simulink model "f1simlu"  (R2026a)
settings: Solver=VariableStepAuto  StopTime=30
values from neighbouring files (symbols this model uses):
  A = 2.2    [vehicleparameter.m]
  Cd = 0.32    [vehicleparameter.m]
  F_drive = 4000    [vehicleparameter.m]
  m = masses(k)    [laptimestudy.m]    (also in runsensitivitystudy 2.m; vehicleparameter.m = 800)
  rho = 1.225    [vehicleparameter.m]
  theta = deg2rad(theta_deg(k))    [roadgradientstudy.m]    (also in vehicleparameter.m = 0)
settings Model: Creator=manoj  LastModifiedBy=manoj

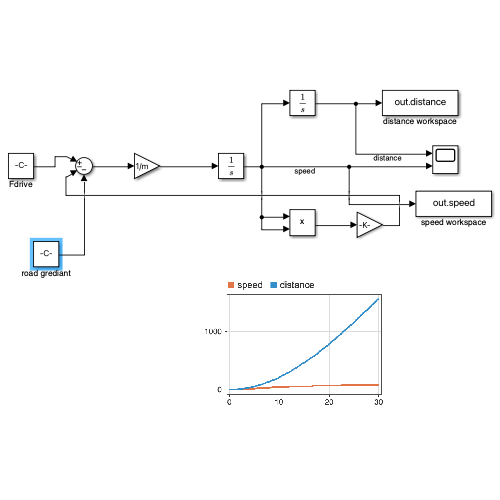
[thumbnail: Simulink's stored preview of the top-level diagram]
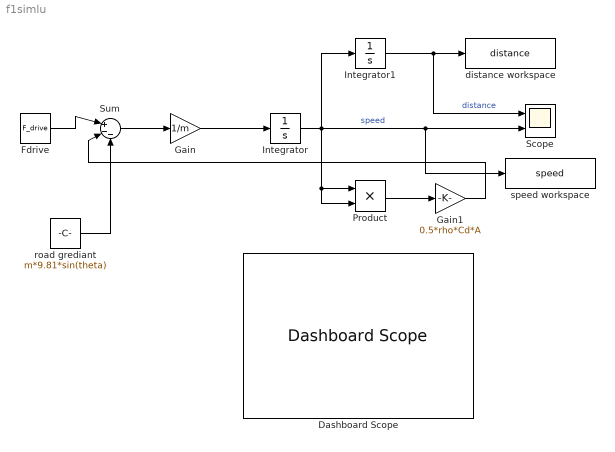
== system f1simlu ==
  Dashboard Scope : DashboardScope  FontColor=[0.0, 0.0, 0.0]
  Fdrive : Constant  Value=F_drive
  Gain : Gain  Gain=1/m
  Gain1 : Gain  Gain=0.5*rho*Cd*A
  Integrator : Integrator
  Integrator1 : Integrator
  Product : Product
  Scope : Scope  NumInputPorts=2
      settings: ActiveDisplayYMinimum=-195.14102866522131  ActiveDisplayYMaximum=1756.2692579869922
  Sum : Sum  Inputs=|+--
  distance workspace : ToWorkspace  VariableName=distance  SaveFormat=Structure With Time  SampleTime=-1
  road grediant : Constant  Value=m*9.81*sin(theta)
  speed workspace : ToWorkspace  VariableName=speed  SaveFormat=Structure With Time  SampleTime=-1
  wires:
  Fdrive/1 -> Sum/1
  Sum/1 -> Gain/1
  Gain/1 -> Integrator/1
  Integrator/1 -> Product/2, Product/1, Integrator1/1, speed workspace/1, Scope/2  "speed"
  Integrator1/1 -> distance workspace/1, Scope/1  "distance"
  Product/1 -> Gain1/1
  Gain1/1 -> Sum/2
  road grediant/1 -> Sum/3
